simulink model "mdl_VD_st5dofModelFriction_ConstantSpeed"  (R2019b)
settings: Solver=ode4  StartTime=0.0  StopTime=50  FixedStep=deltaT  RelTol=1e-4  EnableMultiTasking=on
values from neighbouring files (symbols this model uses):
  friction_coefficient = [0.9, 0.9]    [script_test_mdl_VD_st5dofModel.m]    (also in script_test_mdl_VD_st5dofModelFriction.m; script_test_mdl_VD_st5dofModelFriction_ConstantSpeed.m)
  Period = 3    [script_test_mdl_VD_BicycleModel.m]    (also in script_test_mdl_VD_st5dofModel.m; script_test_mdl_VD_st5dofModelFriction.m; script_test_mdl_VD_st5dofModelFriction_ConstantSpeed.m)
  steering_amplitude = 2*pi/180    (= 0.0349065850399)    [script_test_mdl_VD_st5dofModel.m]    (also in script_test_mdl_VD_st5dofModelFriction.m; script_test_mdl_VD_st5dofModelFriction_ConstantSpeed.m)
undefined symbols (not defined in the file or in its folder): initial, road_properties, vdParam, vehicle
libraries: simulink x5
settings Model: Creator=cbeal  LastModifiedBy=prasa
settings SolverCC: ZeroCrossAlgorithm=Adaptive
settings DataIOCC: SaveFormat=Array  SaveTime=off  ReturnWorkspaceOutputs=off
settings OptimizationCC: ExpressionDepthLimit=2147483647  LifeSpan=inf
settings DebuggingCC: ReadBeforeWriteMsg=DisableAll  WriteAfterWriteMsg=DisableAll  WriteAfterReadMsg=DisableAll  UnderspecifiedInitializationDetection=Classic  MergeDetectMultiDrivingBlocksExec=none  SolverPrmCheckMsg=warning  MultiTaskDSMMsg=none  FcnCallInpInsideContextMsg=warning  StateNameClashWarn=warning  SFUnexpectedBacktrackingDiag=warning  SFNoUnconditionalDefaultTransitionDiag=warning  SFExecutionAtInitializationDiag=none  ArithmeticOperatorsInVariantConditions=warning
settings HardwareCC: ProdBitPerPointer=32  ProdBitPerSizeT=32  ProdBitPerPtrDiffT=32  ProdLargestAtomicFloat=None  ProdIntDivRoundTo=Undefined  ProdEndianess=Unspecified  ProdWordSize=32  ProdHWDeviceType=32-bit Generic
settings ModelReferenceCC: UpdateModelReferenceTargets=IfOutOfDate  PropagateSignalLabelsOutOfModel=off
settings SFSimCC: SFSimEcho=off  SimUseLocalCustomCode=off  CustomCodeUndefinedFunction=UseInterfaceOnly
settings RTWCC: RTWUseLocalCustomCode=off
settings CodeAppCC: StateflowObjectComments=on
settings GRTTargetCC: TargetLangStandard=C89/C90 (ANSI)
settings ConfigComp: CovMetricSettings=dw  CovHtmlReporting=on  CovSaveCumulativeToWorkspaceVar=on  CovSaveSingleToWorkspaceVar=on  CovExternalEMLEnable=off

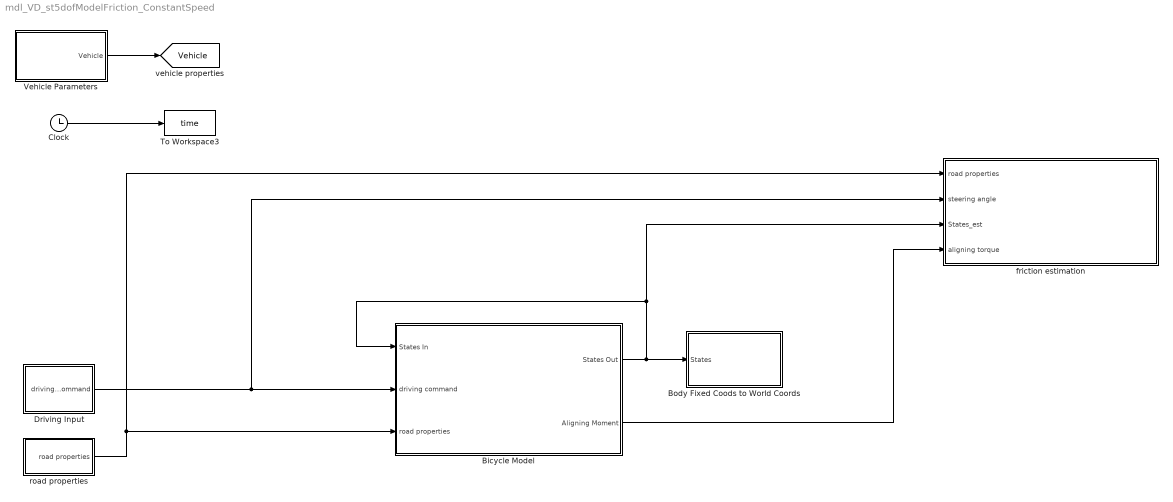
== system mdl_VD_st5dofModelFriction_ConstantSpeed ==
  Bicycle Model : Subsystem
  Body Fixed Coods to World Coords : Subsystem
      mask Display: image('$imagefile'); % Use "Edit Image" on toolstrip to change.
  Clock : Clock
  Driving Input : Subsystem
  To Workspace3 : ToWorkspace  VariableName=time  SampleTime=-1
  Vehicle Parameters : Subsystem  mask{vehicleName='C5 Vette', m=1600, Izz=2500, Iw=1.2, Re=0.32, a=1.3, b=1.3, d=1.5, h_cg=0.42, Ca=[95000; 95000; 110000; 110000], Cx=[65000,65000,65000,65000]}
      mask prompts: vehicleName "Name of Vehicle"; m "Mass"; Izz "Yaw Moment of Inertia"; Iw "Wheel Moment of Inertia"; Re "Wheel Effective Radius"; a "CG-Front Axle Distance"; b "CG-Rear Axle Distance"; d "Track Width"; h_cg "CG height"; Ca "Cornering Stiffnesses (x4)"; Cx "Longitudinal Stiffnesses (x4)"
      mask Display: port_label('output',1,vehicleName)
  friction estimation : Subsystem
  road properties : Subsystem
  tag scope: Vehicle=global
  wires:
  Clock/1 -> To Workspace3/1
  Driving Input/1(driving command) -> friction estimation/2(steering angle), Bicycle Model/2(driving command)
  road properties/1(road properties) -> Bicycle Model/3(road properties), friction estimation/1(road properties)
  Vehicle Parameters/1(Vehicle) -> [Vehicle]
  Bicycle Model/1(States Out) -> Bicycle Model/1(States In), friction estimation/3(States_est), Body Fixed Coods to World Coords/1(States)
  Bicycle Model/2(Aligning Moment) -> friction estimation/4(aligning torque)

== system mdl_VD_st5dofModelFriction_ConstantSpeed/Bicycle Model ==
  States In : Inport
  driving command : Inport  Port=2
  road properties : Inport  Port=3
  Brush Model : Subsystem
  Normal Forces : Subsystem
      mask Display: image('$imagefile'); % Use "Edit Image" on toolstrip to change.
  Slips : Subsystem
      mask Display: image('$imagefile'); % Use "Edit Image" on toolstrip to change.
  Vehicle Body Newtonian Dynamics : Subsystem
      mask Display: image('$imagefile'); % Use "Edit Image" on toolstrip to change.
  States Out : Outport
  Aligning Moment : Outport  Port=2
  wires:
  road properties/1 -> Normal Forces/2(road geometry), Brush Model/3(Road Friction), Vehicle Body Newtonian Dynamics/4(Road Geometry)
  Normal Forces/1(Normal Forces) -> Brush Model/2(Normal Forces)  "Normal Forces"
  States In/1 -> Slips/1(Speeds), Normal Forces/1(accelerations), Vehicle Body Newtonian Dynamics/3(States_IN)
  Vehicle Body Newtonian Dynamics/1(States_Out) -> States Out/1
  Brush Model/1(Aligning Moment) -> Aligning Moment/1
  Slips/1(Slips) -> Brush Model/1(Slips)  "Slips"
  Brush Model/2(Tire Forces) -> Vehicle Body Newtonian Dynamics/1(Tire Forces)
  driving command/1 -> Slips/2(steering angle), Vehicle Body Newtonian Dynamics/2(Driving Command)

== system mdl_VD_st5dofModelFriction_ConstantSpeed/Body Fixed Coods to World Coords ==
  States : Inport
  Bus Creator1 : BusCreator  Inputs=3
  Bus Selector4 : BusSelector  OutputSignals=speeds.Vx,speeds.Vy,speeds.r
  Integrator_East : Integrator  InitialCondition=initial.east
  Integrator_North : Integrator  InitialCondition=initial.north
  Integrator_Psi : Integrator  InitialCondition=initial.heading
  Product{4..7} (4 alike) : Product  SaturateOnIntegerOverflow=on  OutDataTypeStr=Inherit: Same as first input
  Sum : Sum  Inputs=+-  SaturateOnIntegerOverflow=on
  Sum1 : Sum  SaturateOnIntegerOverflow=on
  To Workspace6 : ToWorkspace  VariableName=pose  SampleTime=-1
  Trigonometric Function2 : Trigonometry
  Trigonometric Function3 : Trigonometry  Operator=cos
  wires:
  Bus Creator1/1 -> To Workspace6/1
  Product4/1 -> Sum1/1
  Product6/1 -> Sum/2
  Product7/1 -> Sum1/2
  Trigonometric Function2/1 -> Product4/2, Product6/2
  Integrator_Psi/1 -> Bus Creator1/3, Trigonometric Function3/1, Trigonometric Function2/1  "PSI"
  Sum1/1 -> Integrator_North/1
  Sum/1 -> Integrator_East/1
  Trigonometric Function3/1 -> Product5/2, Product7/2
  Integrator_East/1 -> Bus Creator1/1  "East"
  Product5/1 -> Sum/1
  Integrator_North/1 -> Bus Creator1/2  "North"
  Bus Selector4/1 -> Product4/1, Product5/1  "<Vx>"
  Bus Selector4/3 -> Integrator_Psi/1  "<r>"
  Bus Selector4/2 -> Product7/1, Product6/1  "<Vy>"
  States/1 -> Bus Selector4/1

== system mdl_VD_st5dofModelFriction_ConstantSpeed/Driving Input ==
  Bus Creator1 : BusCreator  Inputs=1
  Mux2 : Mux  Inputs=2
  Product : Product  SaturateOnIntegerOverflow=on  OutDataTypeStr=Inherit: Same as first input
  Rear Steering : Constant  Value=0
  Sine Wave : Sin  Amplitude=steering_amplitude  Frequency=2*pi/Period  SampleTime=0
  Step : Step  Time=0  SampleTime=0
  Step1 : Step  Time=Period  SampleTime=0
  Sum : Sum  Inputs=|+-  SaturateOnIntegerOverflow=on
  To Workspace3 : ToWorkspace  VariableName=delta  SampleTime=-1
  driving command : Outport
  wires:
  Mux2/1 -> To Workspace3/1, Bus Creator1/1  "steering angle"
  Bus Creator1/1 -> driving command/1
  Step1/1 -> Sum/2
  Sine Wave/1 -> Product/2
  Sum/1 -> Product/1
  Product/1 -> Mux2/1
  Step/1 -> Sum/1
  Rear Steering/1 -> Mux2/2

== system mdl_VD_st5dofModelFriction_ConstantSpeed/Vehicle Parameters ==
  Bus Creator1 : BusCreator  Inputs=11
  Constant : Constant  Value=vehicle.m
  Constant1 : Constant  Value=vehicle.Izz
  Constant13 : Constant  Value=vehicle.Re
  Constant14 : Constant  Value=vehicle.h_cg
  Constant2 : Constant  Value=vehicle.L
  Constant3 : Constant  Value=vehicle.d
  Constant4 : Constant  Value=vehicle.b
  Constant5 : Constant  Value=vehicle.a
  Constant7 : Constant  Value=vehicle.Ca
  Constant8 : Constant  Value=vehicle.Cx
  Constant9 : Constant  Value=vehicle.Iw
  Vehicle : Outport
  wires:
  Bus Creator1/1 -> Vehicle/1
  Constant/1 -> Bus Creator1/1  "m"
  Constant1/1 -> Bus Creator1/2  "Izz"
  Constant9/1 -> Bus Creator1/3  "Iw"
  Constant13/1 -> Bus Creator1/4  "Re"
  Constant2/1 -> Bus Creator1/6  "L"
  Constant14/1 -> Bus Creator1/9  "h_cg"
  Constant7/1 -> Bus Creator1/10  "Ca"
  Constant8/1 -> Bus Creator1/11  "Cx"
  Constant5/1 -> Bus Creator1/5  "a"
  Constant3/1 -> Bus Creator1/8  "d"
  Constant4/1 -> Bus Creator1/7  "b"

== system mdl_VD_st5dofModelFriction_ConstantSpeed/friction estimation ==
  road properties : Inport
  steering angle : Inport  Port=2
  States_est : Inport  Port=3
  aligning torque : Inport  Port=4
  Bus Selector1 : BusSelector  OutputSignals=road friction,road geometry
  Bus Selector2 : BusSelector  OutputSignals=steering angle
  Friction Coefficients Estimate : Subsystem
  Noise Models : Subsystem
  Normal Forces : Subsystem
      mask Display: image('$imagefile'); % Use "Edit Image" on toolstrip to change.
  Slip Angle : Subsystem
      mask Display: image('$imagefile'); % Use "Edit Image" on toolstrip to change.
  To Workspace1 : ToWorkspace  VariableName=friction_coefficients_estimate  SampleTime=-1
  fric est Calculate Xis : Subsystem
  wires:
  States_est/1 -> Noise Models/1(" States")
  Bus Selector2/1 -> Slip Angle/2(delta)  "<steering angle>"
  aligning torque/1 -> Friction Coefficients Estimate/1(Mz)
  fric est Calculate Xis/1(fric est coefficients) -> Friction Coefficients Estimate/2(fric est coefficients)
  Normal Forces/1(Normal Forces) -> Friction Coefficients Estimate/3(fric est Normal Forces)
  Bus Selector1/2 -> Normal Forces/2(road geometry)  "<road geometry>"
  Friction Coefficients Estimate/1(friction coefficients Estimate) -> To Workspace1/1  "friction_coeffs_estimate"
  Bus Selector1/1 -> fric est Calculate Xis/2(friction coefficients)  "<road friction>"
  road properties/1 -> Bus Selector1/1
  Slip Angle/1(Slip Angles) -> fric est Calculate Xis/1(Slip Angles est)
  Noise Models/1(Speeds) -> Slip Angle/1(Speeds)
  steering angle/1 -> Bus Selector2/1
  Noise Models/2(Accelerations) -> Normal Forces/1(accelerations)

== system mdl_VD_st5dofModelFriction_ConstantSpeed/road properties ==
  Bus Creator1 : BusCreator  Inputs=3
  Bus Creator2 : BusCreator  Inputs=2
  Constant1 : Constant  Value=road_properties.grade
  Constant19 : Constant  Value=road_properties.bank_angle
  Constant3 : Constant  Value=0
  Constant4 : Constant  Value=friction_coefficient
  road properties : Outport
  wires:
  Constant1/1 -> Bus Creator1/2  "grade"
  Constant19/1 -> Bus Creator1/1  "banking angle"
  Constant3/1 -> Bus Creator1/3  "Curvature"
  Constant4/1 -> Bus Creator2/2  "road friction"
  Bus Creator2/1 -> road properties/1  "road properties"
  Bus Creator1/1 -> Bus Creator2/1  "road geometry"

== system mdl_VD_st5dofModelFriction_ConstantSpeed/Bicycle Model/Brush Model ==
  Slips : Inport
  Normal Forces : Inport  Port=2
  Road Friction : Inport  Port=3
  Aligning Moment_Brush Model : Subsystem
      mask Display: image('$imagefile'); % Use "Edit Image" on toolstrip to change.
  Tire Forces_Brush Model : Subsystem
      mask Display: image('$imagefile'); % Use "Edit Image" on toolstrip to change.
  Aligning Moment : Outport
  Tire Forces : Outport  Port=2
  wires:
  Road Friction/1 -> Aligning Moment_Brush Model/3(Friction Coefficients), Tire Forces_Brush Model/3(road friction)
  Tire Forces_Brush Model/1(Tire Forces) -> Tire Forces/1  "Tire Forces"
  Aligning Moment_Brush Model/1(Aligning Moment) -> Aligning Moment/1  "Aligning Moment"
  Normal Forces/1 -> Tire Forces_Brush Model/2(Normal Forces), Aligning Moment_Brush Model/2(Normal Forces)
  Slips/1 -> Tire Forces_Brush Model/1(Slips), Aligning Moment_Brush Model/1(Slip Angles)

== system mdl_VD_st5dofModelFriction_ConstantSpeed/Bicycle Model/Normal Forces ==
  accelerations : Inport
  road geometry : Inport  Port=2
  Front : Sum  Inputs=+-
  Mux : Mux  Inputs=2
  Normal Force Longitudinal Transfer : Subsystem
      mask Display: image('$imagefile'); % Use "Edit Image" on toolstrip to change.
  Normal Force Static : Subsystem
  Rear : Sum
  Normal Forces : Outport
  wires:
  Mux/1 -> Normal Forces/1
  Front/1 -> Mux/1
  Rear/1 -> Mux/2
  Normal Force Static/2(Static Rear) -> Rear/1
  Normal Force Static/1(Static Front) -> Front/1
  road geometry/1 -> Normal Force Static/1(road geometry)
  Normal Force Longitudinal Transfer/1(Long Transfer) -> Front/2, Rear/2
  accelerations/1 -> Normal Force Longitudinal Transfer/1(Accelerations)

== system mdl_VD_st5dofModelFriction_ConstantSpeed/Bicycle Model/Slips ==
  Speeds : Inport
  steering angle : Inport  Port=2
  Bus Creator : BusCreator  Inputs=2
  Bus Selector1 : BusSelector  OutputSignals=speeds
  Bus Selector2 : BusSelector  OutputSignals=steering angle
  Slip Angle : Subsystem
      mask Display: image('$imagefile'); % Use "Edit Image" on toolstrip to change.
  To Workspace : ToWorkspace  VariableName=alpha  SampleTime=-1
  To Workspace4 : ToWorkspace  VariableName=kappa  SampleTime=-1
  Wheel Slip Ratio : Subsystem
      mask Display: image('$imagefile'); % Use "Edit Image" on toolstrip to change.
  Slips : Outport
  wires:
  Slip Angle/1(Slip Angles) -> Bus Creator/1, To Workspace/1  "Slip Angles"
  Bus Selector2/1 -> Wheel Slip Ratio/1(delta), Slip Angle/2(delta)  "<steering angle>"
  Wheel Slip Ratio/1(Wheel Slips) -> To Workspace4/1, Bus Creator/2  "Wheel Slips"
  Bus Selector1/1 -> Slip Angle/1(Speeds), Wheel Slip Ratio/2(Speeds)  "<speeds>"
  Bus Creator/1 -> Slips/1
  Speeds/1 -> Bus Selector1/1
  steering angle/1 -> Bus Selector2/1

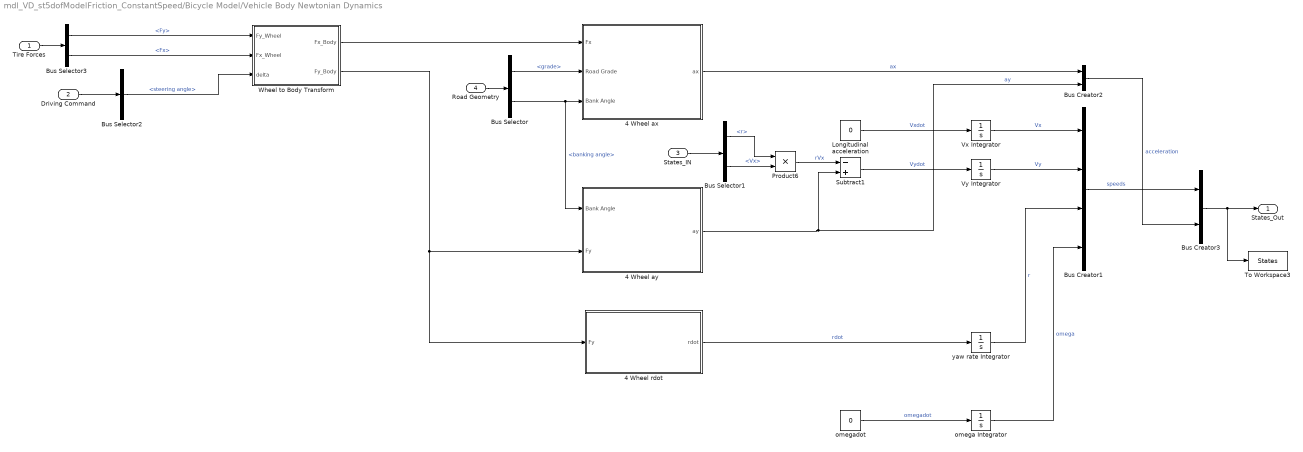
== system mdl_VD_st5dofModelFriction_ConstantSpeed/Bicycle Model/Vehicle Body Newtonian Dynamics ==
  Tire Forces : Inport
  Driving Command : Inport  Port=2
  States_IN : Inport  Port=3
  Road Geometry : Inport  Port=4
  4 Wheel ax : Subsystem
  4 Wheel ay : Subsystem
  4 Wheel rdot : Subsystem
  Bus Creator1 : BusCreator  Inputs=4
  Bus Creator2 : BusCreator  Inputs=2
  Bus Creator3 : BusCreator  Inputs=2
  Bus Selector : BusSelector  OutputSignals=road geometry.grade,road geometry.banking angle
  Bus Selector1 : BusSelector  OutputSignals=speeds.r,speeds.Vx
  Bus Selector2 : BusSelector  OutputSignals=steering angle
  Bus Selector3 : BusSelector  OutputSignals=Fy,Fx
  Longitudinal acceleration : Constant  Value=0
  Product6 : Product  RndMeth=Zero
  Subtract1 : Sum  Inputs=-+
  To Workspace3 : ToWorkspace  VariableName=States  SampleTime=-1
  Vx Integrator : Integrator  InitialCondition=initial.longitudinalSpeed
  Vy Integrator : Integrator
  Wheel to Body Transform : Subsystem
  omega Integrator : Integrator  InitialCondition=initial.wheelSpeeds
  omegadot : Constant  Value=0
  yaw rate Integrator : Integrator
  States_Out : Outport
  wires:
  omegadot/1 -> omega Integrator/1  "omegadot"
  yaw rate Integrator/1 -> Bus Creator1/3  "r"
  Vy Integrator/1 -> Bus Creator1/2  "Vy"
  Vx Integrator/1 -> Bus Creator1/1  "Vx"
  omega Integrator/1 -> Bus Creator1/4  "omega"
  Bus Creator2/1 -> Bus Creator3/2  "acceleration"
  Product6/1 -> Subtract1/1  "rVx"
  Longitudinal acceleration/1 -> Vx Integrator/1  "Vxdot"
  Bus Selector/1 -> 4 Wheel ax/2(Road Grade)  "<grade>"
  Wheel to Body Transform/2(Fy_Body) -> 4 Wheel rdot/1(Fy), 4 Wheel ay/2(Fy)
  Wheel to Body Transform/1(Fx_Body) -> 4 Wheel ax/1("Fx ")
  4 Wheel rdot/1(rdot) -> yaw rate Integrator/1  "rdot"
  4 Wheel ay/1(ay) -> Bus Creator2/2, Subtract1/2  "ay"
  4 Wheel ax/1(ax) -> Bus Creator2/1  "ax"
  Bus Creator1/1 -> Bus Creator3/1  "speeds"
  Bus Selector/2 -> 4 Wheel ay/1(Bank Angle), 4 Wheel ax/3(Bank Angle)  "<banking angle>"
  Road Geometry/1 -> Bus Selector/1
  Bus Selector2/1 -> Wheel to Body Transform/3(delta)  "<steering angle>"
  States_IN/1 -> Bus Selector1/1
  Bus Selector1/2 -> Product6/2  "<Vx>"
  Bus Selector1/1 -> Product6/1  "<r>"
  Tire Forces/1 -> Bus Selector3/1
  Bus Selector3/2 -> Wheel to Body Transform/2(Fx_Wheel)  "<Fx>"
  Bus Selector3/1 -> Wheel to Body Transform/1(Fy_Wheel)  "<Fy>"
  Driving Command/1 -> Bus Selector2/1
  Bus Creator3/1 -> To Workspace3/1, States_Out/1
  Subtract1/1 -> Vy Integrator/1  "Vydot"

== system mdl_VD_st5dofModelFriction_ConstantSpeed/friction estimation/Friction Coefficients Estimate ==
  Mz : Inport
  fric est coefficients : Inport  Port=2
  fric est Normal Forces : Inport  Port=3
  Demux1 : Demux
  Divide : Product  Inputs=*/
  Estimate Friction Force : M-S-Function  FunctionName=sfcn_estimateFrictionForce_Bicycle
  To Workspace5 : ToWorkspace  VariableName=frictionalForce_est  SampleTime=-1
  friction coefficients Estimate : Outport
  wires:
  fric est coefficients/1 -> Demux1/1
  Estimate Friction Force/1 -> Divide/1, To Workspace5/1
  Mz/1 -> Estimate Friction Force/1
  Demux1/1 -> Estimate Friction Force/2  "Xi1"
  Demux1/2 -> Estimate Friction Force/3  "Xi2"
  Demux1/3 -> Estimate Friction Force/4  "Xi3"
  Demux1/4 -> Estimate Friction Force/5  "Xi4"
  fric est Normal Forces/1 -> Divide/2
  Divide/1 -> friction coefficients Estimate/1

== system mdl_VD_st5dofModelFriction_ConstantSpeed/friction estimation/Noise Models ==
  " States" : Inport
  Bus Creator1 : BusCreator  Inputs=3
  Bus Creator2 : BusCreator  Inputs=2
  Bus Creator3 : BusCreator  Inputs=2
  Bus Selector1 : BusSelector  OutputSignals=acceleration,speeds
  Bus Selector2 : BusSelector  OutputSignals=Vx,Vy,r
  Bus Selector3 : BusSelector  OutputSignals=ax,ay
  GPS Noise Function : MATLAB Function  TreatAsAtomicUnit=on
  IMU Noise Function : MATLAB Function  TreatAsAtomicUnit=on
  Sampling Time : Constant  Value=vdParam.sampling_time_gps
  Sampling Time1 : Constant  Value=vdParam.sampling_time_imu
  Speeds : Outport
  Accelerations : Outport  Port=2
  wires:
  Bus Selector2/3 -> GPS Noise Function/3(r)  "<r>"
  Bus Selector1/2 -> Bus Selector2/1  "<speeds>"
  Bus Selector2/2 -> GPS Noise Function/2(v_y)  "<Vy>"
  Bus Selector2/1 -> GPS Noise Function/1(v_x)  "<Vx>"
  Bus Creator1/1 -> Bus Creator3/2, Speeds/1  "speeds"
  Bus Selector3/1 -> IMU Noise Function/1(a_x)  "<ax>"
  Bus Selector3/2 -> IMU Noise Function/2(a_y)  "<ay>"
  Bus Selector1/1 -> Bus Selector3/1  "<acceleration>"
  GPS Noise Function/3(r_out) -> Bus Creator1/3  "r"
  Bus Creator2/1 -> Bus Creator3/1  "acceleration"
  Sampling Time/1 -> GPS Noise Function/4(sampling_time)
  GPS Noise Function/1(v_x_out) -> Bus Creator1/1  "Vx"
  GPS Noise Function/2(v_y_out) -> Bus Creator1/2  "Vy"
  IMU Noise Function/2(a_y_out) -> Bus Creator2/2  "ay"
  IMU Noise Function/1(a_x_out) -> Bus Creator2/1  "ax"
  Sampling Time1/1 -> IMU Noise Function/3(sampling_time)
  " States"/1 -> Bus Selector1/1
  Bus Creator3/1 -> Accelerations/1

== system mdl_VD_st5dofModelFriction_ConstantSpeed/friction estimation/Normal Forces ==
  accelerations : Inport
  road geometry : Inport  Port=2
  Front : Sum  Inputs=+-
  Mux : Mux  Inputs=2
  Normal Force Longitudinal Transfer : Subsystem
      mask Display: image('$imagefile'); % Use "Edit Image" on toolstrip to change.
  Normal Force Static : Subsystem
  Rear : Sum
  Normal Forces : Outport
  wires:
  Mux/1 -> Normal Forces/1
  Front/1 -> Mux/1
  Rear/1 -> Mux/2
  Normal Force Static/2(Static Rear) -> Rear/1
  Normal Force Static/1(Static Front) -> Front/1
  road geometry/1 -> Normal Force Static/1(road geometry)
  Normal Force Longitudinal Transfer/1(Long Transfer) -> Front/2, Rear/2
  accelerations/1 -> Normal Force Longitudinal Transfer/1(Accelerations)

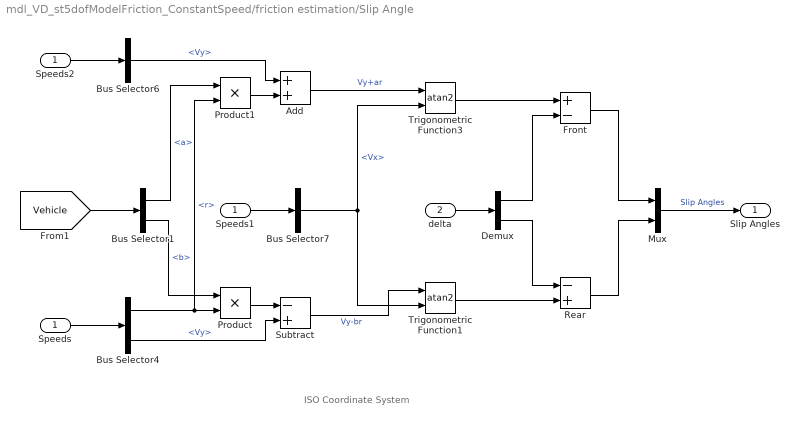
== system mdl_VD_st5dofModelFriction_ConstantSpeed/friction estimation/Slip Angle ==
  note: ISO Coordinate System
  Speeds : Inport
  delta : Inport  Port=2
  Add : Sum
  Bus Selector1 : BusSelector  OutputSignals=a,b
  Bus Selector4 : BusSelector  OutputSignals=r,Vy
  Bus Selector6 : BusSelector  OutputSignals=Vy
  Bus Selector7 : BusSelector  OutputSignals=Vx
  Demux : Demux  Outputs=2
  Front : Sum  Inputs=+-
  Mux : Mux  Inputs=2
  Product : Product  RndMeth=Zero
  Product1 : Product  RndMeth=Zero
  Rear : Sum  Inputs=-+
  Speeds1 : InportShadow
  Speeds2 : InportShadow
  Subtract : Sum  Inputs=-+
  Trigonometric Function1 : Trigonometry  Operator=atan2
  Trigonometric Function3 : Trigonometry  Operator=atan2
  Slip Angles : Outport
  wires:
  Speeds1/1 -> Bus Selector7/1
  Bus Selector4/1 -> Product1/2, Product/2  "<r>"
  Demux/1 -> Front/2
  Subtract/1 -> Trigonometric Function1/1  "Vy-br"
  Trigonometric Function1/1 -> Rear/2
  delta/1 -> Demux/1
  Rear/1 -> Mux/2
  Demux/2 -> Rear/1
  Add/1 -> Trigonometric Function3/1  "Vy+ar"
  [Vehicle] -> Bus Selector1/1
  Product/1 -> Subtract/1
  Mux/1 -> Slip Angles/1  "Slip Angles"
  Bus Selector1/2 -> Product/1  "<b>"
  Front/1 -> Mux/1
  Bus Selector1/1 -> Product1/1  "<a>"
  Trigonometric Function3/1 -> Front/1
  Product1/1 -> Add/2
  Bus Selector7/1 -> Trigonometric Function3/2, Trigonometric Function1/2  "<Vx>"
  Speeds2/1 -> Bus Selector6/1
  Bus Selector4/2 -> Subtract/2  "<Vy>"
  Bus Selector6/1 -> Add/1  "<Vy>"
  Speeds/1 -> Bus Selector4/1

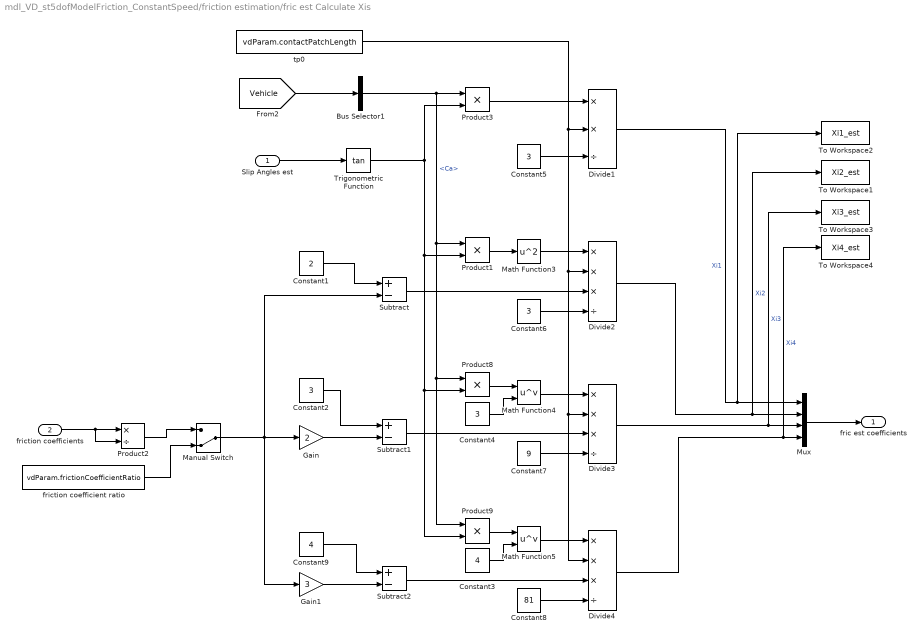
== system mdl_VD_st5dofModelFriction_ConstantSpeed/friction estimation/fric est Calculate Xis ==
  Slip Angles est : Inport
  friction coefficients : Inport  Port=2
  Bus Selector1 : BusSelector  OutputSignals=Ca
  Constant1 : Constant  Value=2
  Constant{2,4..6} (4 alike) : Constant  Value=3
  Constant3 : Constant  Value=4
  Constant7 : Constant  Value=9
  Constant8 : Constant  Value=81
  Constant9 : Constant  Value=4
  Divide1 : Product  Inputs=**/
  Divide2 : Product  Inputs=***/
  Divide3 : Product  Inputs=***/
  Divide4 : Product  Inputs=***/
  Gain : Gain  Gain=2
  Gain1 : Gain  Gain=3
  Manual Switch : ManualSwitch  CurrentSetting=0
  Math Function3 : Math  Operator=square  SaturateOnIntegerOverflow=on
  Math Function4 : Math  Operator=pow  SignedPower=off  SaturateOnIntegerOverflow=on
  Math Function5 : Math  Operator=pow  SignedPower=off  SaturateOnIntegerOverflow=on
  Mux : Mux
  Product{1,3,8..9} (4 alike) : Product  RndMeth=Zero
  Product2 : Product  Inputs=*/  RndMeth=Zero
  Subtract : Sum  Inputs=+-
  Subtract1 : Sum  Inputs=+-
  Subtract2 : Sum  Inputs=+-
  To Workspace1 : ToWorkspace  VariableName=Xi2_est  SampleTime=-1
  To Workspace2 : ToWorkspace  VariableName=Xi1_est  SampleTime=-1
  To Workspace3 : ToWorkspace  VariableName=Xi3_est  SampleTime=-1
  To Workspace4 : ToWorkspace  VariableName=Xi4_est  SampleTime=-1
  Trigonometric Function : Trigonometry  Operator=tan
  friction coefficient ratio : Constant  Value=vdParam.frictionCoefficientRatio
  tp0 : Constant  Value=vdParam.contactPatchLength
  fric est coefficients : Outport
  wires:
  Mux/1 -> fric est coefficients/1
  Trigonometric Function/1 -> Product1/2, Product8/2, Product9/2, Product3/2
  tp0/1 -> Divide4/2, Divide3/2, Divide2/2, Divide1/2
  Bus Selector1/1 -> Product9/1, Product8/1, Product1/1, Product3/1  "<Ca>"
  Constant3/1 -> Math Function5/2
  Constant4/1 -> Math Function4/2
  Math Function3/1 -> Divide2/1
  Product1/1 -> Math Function3/1
  [Vehicle] -> Bus Selector1/1
  Math Function4/1 -> Divide3/1
  Constant5/1 -> Divide1/3
  Slip Angles est/1 -> Trigonometric Function/1
  Math Function5/1 -> Divide4/1
  Product8/1 -> Math Function4/1
  Product9/1 -> Math Function5/1
  Constant7/1 -> Divide3/4
  Product3/1 -> Divide1/1
  Subtract1/1 -> Divide3/3
  Constant1/1 -> Subtract/1
  Constant2/1 -> Subtract1/1
  Manual Switch/1 -> Gain1/1, Subtract/2, Gain/1
  Gain/1 -> Subtract1/2
  Constant9/1 -> Subtract2/1
  Gain1/1 -> Subtract2/2
  Constant6/1 -> Divide2/4
  Subtract/1 -> Divide2/3
  Constant8/1 -> Divide4/4
  Subtract2/1 -> Divide4/3
  Divide1/1 -> To Workspace2/1, Mux/1  "Xi1"
  Divide4/1 -> To Workspace4/1, Mux/4  "Xi4"
  Divide2/1 -> To Workspace1/1, Mux/2  "Xi2"
  Divide3/1 -> To Workspace3/1, Mux/3  "Xi3"
  friction coefficients/1 -> Product2/2, Product2/1
  Product2/1 -> Manual Switch/1
  friction coefficient ratio/1 -> Manual Switch/2

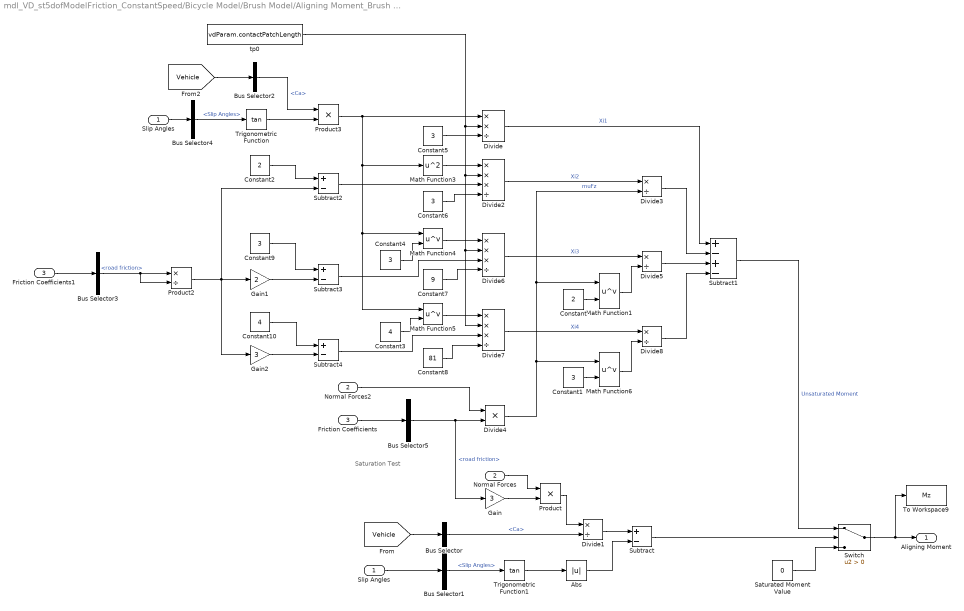
== system mdl_VD_st5dofModelFriction_ConstantSpeed/Bicycle Model/Brush Model/Aligning Moment_Brush Model ==
  note: Saturation Test
  Slip Angles : Inport
  Normal Forces : Inport  Port=2
  Friction Coefficients : Inport  Port=3
  Abs : Abs  ZeroCross=off
  Bus Selector : BusSelector  OutputSignals=Ca
  Bus Selector1 : BusSelector  OutputSignals=Slip Angles
  Bus Selector2 : BusSelector  OutputSignals=Ca
  Bus Selector3 : BusSelector  OutputSignals=road friction
  Bus Selector4 : BusSelector  OutputSignals=Slip Angles
  Bus Selector5 : BusSelector  OutputSignals=road friction
  Constant : Constant  Value=2
  Constant{1,4..6,9} (5 alike) : Constant  Value=3
  Constant10 : Constant  Value=4
  Constant2 : Constant  Value=2
  Constant3 : Constant  Value=4
  Constant7 : Constant  Value=9
  Constant8 : Constant  Value=81
  Divide : Product  Inputs=**/
  Divide{1,3,5,8} (4 alike) : Product  Inputs=*/
  Divide2 : Product  Inputs=***/
  Divide4 : Product
  Divide6 : Product  Inputs=***/
  Divide7 : Product  Inputs=***/
  Friction Coefficients1 : InportShadow  Port=3
  Gain : Gain  Gain=3
  Gain1 : Gain  Gain=2
  Gain2 : Gain  Gain=3
  Math Function{1,4..6} (4 alike) : Math  Operator=pow  SignedPower=off  SaturateOnIntegerOverflow=on
  Math Function3 : Math  Operator=square  SaturateOnIntegerOverflow=on
  Normal Forces2 : InportShadow  Port=2
  Product : Product  RndMeth=Zero
  Product2 : Product  Inputs=*/  RndMeth=Zero
  Product3 : Product  RndMeth=Zero
  Saturated Moment Value : Constant  Value=0
  "Slip Angles " : InportShadow
  Subtract{,2..4} (4 alike) : Sum  Inputs=+-
  Subtract1 : Sum  Inputs=+-+-
  Switch : Switch  Criteria=u2 > Threshold
  To Workspace9 : ToWorkspace  VariableName=Mz  SampleTime=-1
  Trigonometric Function : Trigonometry  Operator=tan
  Trigonometric Function1 : Trigonometry  Operator=tan
  tp0 : Constant  Value=vdParam.contactPatchLength
  Aligning Moment : Outport  VectorParamsAs1DForOutWhenUnconnected=off
  wires:
  Product/1 -> Divide1/1
  Switch/1 -> To Workspace9/1, Aligning Moment/1
  Normal Forces2/1 -> Divide4/1
  Abs/1 -> Subtract/2
  Subtract/1 -> Switch/2
  Saturated Moment Value/1 -> Switch/3
  Bus Selector/1 -> Divide1/2  "<Ca>"
  [Vehicle] -> Bus Selector/1
  Divide1/1 -> Subtract/1
  Normal Forces/1 -> Product/1
  Gain/1 -> Product/2
  Trigonometric Function1/1 -> Abs/1
  Slip Angles/1 -> Bus Selector4/1
  Subtract1/1 -> Switch/1  "Unsaturated Moment"
  "Slip Angles "/1 -> Bus Selector1/1
  Divide4/1 -> Divide3/2, Math Function1/1, Math Function6/1  "muFz"
  Constant/1 -> Math Function1/2
  [Vehicle] -> Bus Selector2/1
  Bus Selector2/1 -> Product3/1  "<Ca>"
  Constant3/1 -> Math Function5/2
  Constant4/1 -> Math Function4/2
  Trigonometric Function/1 -> Product3/2
  Product3/1 -> Math Function3/1, Math Function4/1, Math Function5/1, Divide/1
  tp0/1 -> Divide/2, Divide2/2, Divide7/2, Divide6/2
  Constant5/1 -> Divide/3
  Math Function3/1 -> Divide2/1
  Constant7/1 -> Divide6/4
  Math Function4/1 -> Divide6/1
  Math Function5/1 -> Divide7/1
  Constant6/1 -> Divide2/4
  Constant8/1 -> Divide7/4
  Divide3/1 -> Subtract1/2
  Constant1/1 -> Math Function6/2
  Divide8/1 -> Subtract1/4
  Divide5/1 -> Subtract1/3
  Math Function6/1 -> Divide8/2
  Math Function1/1 -> Divide5/2
  Bus Selector5/1 -> Gain/1, Divide4/2  "<road friction>"
  Divide/1 -> Subtract1/1  "Xi1"
  Divide7/1 -> Divide8/1  "Xi4"
  Divide2/1 -> Divide3/1  "Xi2"
  Divide6/1 -> Divide5/1  "Xi3"
  Gain2/1 -> Subtract4/2
  Product2/1 -> Gain2/1, Subtract2/2, Gain1/1
  Constant9/1 -> Subtract3/1
  Subtract3/1 -> Divide6/3
  Constant10/1 -> Subtract4/1
  Constant2/1 -> Subtract2/1
  Subtract2/1 -> Divide2/3
  Subtract4/1 -> Divide7/3
  Gain1/1 -> Subtract3/2
  Bus Selector4/1 -> Trigonometric Function/1  "<Slip Angles>"
  Bus Selector1/1 -> Trigonometric Function1/1  "<Slip Angles>"
  Bus Selector3/1 -> Product2/2, Product2/1  "<road friction>"
  Friction Coefficients1/1 -> Bus Selector3/1
  Friction Coefficients/1 -> Bus Selector5/1

== system mdl_VD_st5dofModelFriction_ConstantSpeed/Bicycle Model/Brush Model/Tire Forces_Brush Model ==
  note: ISO Coordinate System
  note: [1] J. Svendenius, “Tire Modeling and Friction Estimation,” Control , p. 194, 2007. chapter2.4 and chapter4
      | [2] M. Kissai et al. , “A new linear tire model with varying parameters To cite this version : HAL Id : hal-01690792 A New Linear Tire Model With Varying Parameters,” 2018.
  Slips : Inport
  Normal Forces : Inport  Port=2
  road friction : Inport  Port=3
  Bus Selector2 : BusSelector  OutputSignals=road friction
  Constant3 : Constant
  Switch1 : Switch  Threshold=1  ZeroCross=off
  Wheel Forces : Subsystem
  tire slip : Subsystem
  Tire Forces : Outport
  wires:
  tire slip/1(sigma_x) -> Wheel Forces/3(sigma_x)
  Normal Forces/1 -> tire slip/2(normal force), Wheel Forces/2(normal force)
  tire slip/4(Psi_Tire) -> Switch1/3, Switch1/2
  tire slip/2(sigma_y) -> Wheel Forces/4(sigma_y)
  tire slip/3(sigma) -> Wheel Forces/5(sigma)
  Bus Selector2/1 -> Wheel Forces/1(sliding friction), tire slip/1(peak friction)  "<road friction>"
  Wheel Forces/1(Tire Forces) -> Tire Forces/1
  Constant3/1 -> Switch1/1  "Pure Sliding"
  Switch1/1 -> Wheel Forces/6(Psi_Tire)
  Slips/1 -> tire slip/3(Slips)
  road friction/1 -> Bus Selector2/1

== system mdl_VD_st5dofModelFriction_ConstantSpeed/Bicycle Model/Normal Forces/Normal Force Longitudinal Transfer ==
  Accelerations : Inport
  Bus Selector2 : BusSelector  OutputSignals=m,L,h_cg
  Bus Selector3 : BusSelector  OutputSignals=acceleration.ax
  Compare To Constant : simulink/Logic and Bit Operations/Compare To Constant  relop===  const=1  OutDataTypeStr=boolean
  Constant : Constant  Value=vdParam.longitudinalTransfer
  Delay : Delay  DelayLength=1  InitialCondition=0
  Divide1 : Product  Inputs=/*
  Product1 : Product  RndMeth=Zero
  Product2 : Product  RndMeth=Zero
  Product3 : Product  RndMeth=Zero
  Long Transfer : Outport
  wires:
  Bus Selector2/2 -> Divide1/1  "<L>"
  Product3/1 -> Product1/1
  Bus Selector2/3 -> Divide1/2  "<h_cg>"
  Divide1/1 -> Product1/2
  [Vehicle] -> Bus Selector2/1
  Bus Selector2/1 -> Product2/2  "<m>"
  Delay/1 -> Product2/1
  Product2/1 -> Product3/2
  Product1/1 -> Long Transfer/1
  Accelerations/1 -> Bus Selector3/1
  Compare To Constant/1 -> Product3/1
  Constant/1 -> Compare To Constant/1
  Bus Selector3/1 -> Delay/1  "<ax>"

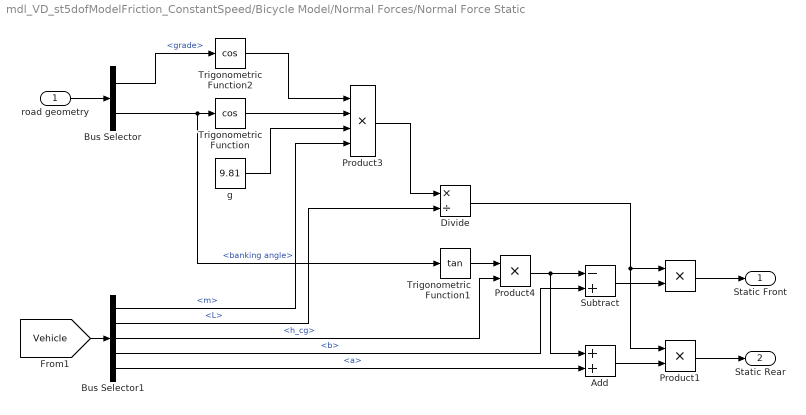
== system mdl_VD_st5dofModelFriction_ConstantSpeed/Bicycle Model/Normal Forces/Normal Force Static ==
  road geometry : Inport
  " " : Product  RndMeth=Zero
  Add : Sum
  Bus Selector : BusSelector  OutputSignals=road geometry.grade,road geometry.banking angle
  Bus Selector1 : BusSelector  OutputSignals=m,L,h_cg,b,a
  Divide : Product  Inputs=*/
  Product1 : Product  RndMeth=Zero
  Product3 : Product  Inputs=4  RndMeth=Zero
  Product4 : Product  RndMeth=Zero
  Subtract : Sum  Inputs=-+
  Trigonometric Function : Trigonometry  Operator=cos
  Trigonometric Function1 : Trigonometry  Operator=tan
  Trigonometric Function2 : Trigonometry  Operator=cos
  g : Constant  Value=9.81
  Static Front : Outport
  Static Rear : Outport  Port=2
  wires:
  Product4/1 -> Add/1, Subtract/1
  Add/1 -> Product1/2
  g/1 -> Product3/3
  [Vehicle] -> Bus Selector1/1
  Bus Selector1/4 -> Subtract/2  "<b>"
  Product3/1 -> Divide/1
  Bus Selector1/1 -> Product3/4  "<m>"
  Trigonometric Function/1 -> Product3/2
  Bus Selector1/5 -> Add/2  "<a>"
  Bus Selector1/3 -> Product4/2  "<h_cg>"
  Trigonometric Function1/1 -> Product4/1
  Divide/1 -> Product1/1, " "/1
  Bus Selector/2 -> Trigonometric Function1/1, Trigonometric Function/1  "<banking angle>"
  Bus Selector1/2 -> Divide/2  "<L>"
  Subtract/1 -> " "/2
  road geometry/1 -> Bus Selector/1
  Product1/1 -> Static Rear/1
  " "/1 -> Static Front/1
  Trigonometric Function2/1 -> Product3/1
  Bus Selector/1 -> Trigonometric Function2/1  "<grade>"

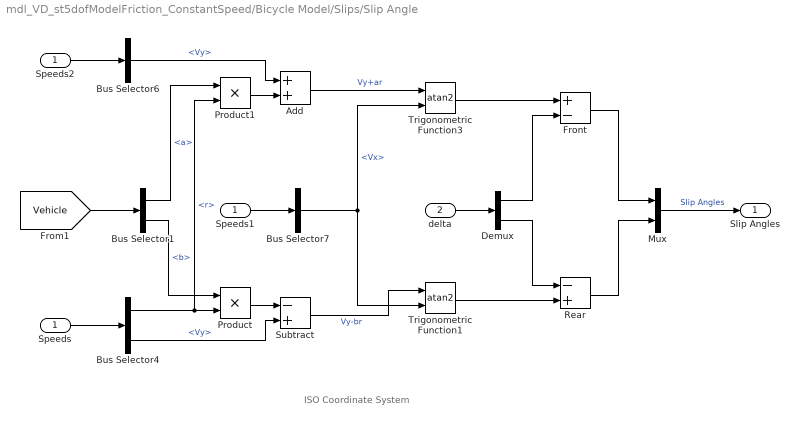
== system mdl_VD_st5dofModelFriction_ConstantSpeed/Bicycle Model/Slips/Slip Angle ==
  note: ISO Coordinate System
  Speeds : Inport
  delta : Inport  Port=2
  Add : Sum
  Bus Selector1 : BusSelector  OutputSignals=a,b
  Bus Selector4 : BusSelector  OutputSignals=r,Vy
  Bus Selector6 : BusSelector  OutputSignals=Vy
  Bus Selector7 : BusSelector  OutputSignals=Vx
  Demux : Demux  Outputs=2
  Front : Sum  Inputs=+-
  Mux : Mux  Inputs=2
  Product : Product  RndMeth=Zero
  Product1 : Product  RndMeth=Zero
  Rear : Sum  Inputs=-+
  Speeds1 : InportShadow
  Speeds2 : InportShadow
  Subtract : Sum  Inputs=-+
  Trigonometric Function1 : Trigonometry  Operator=atan2
  Trigonometric Function3 : Trigonometry  Operator=atan2
  Slip Angles : Outport
  wires:
  Speeds1/1 -> Bus Selector7/1
  Bus Selector4/1 -> Product1/2, Product/2  "<r>"
  Demux/1 -> Front/2
  Subtract/1 -> Trigonometric Function1/1  "Vy-br"
  Trigonometric Function1/1 -> Rear/2
  delta/1 -> Demux/1
  Rear/1 -> Mux/2
  Demux/2 -> Rear/1
  Add/1 -> Trigonometric Function3/1  "Vy+ar"
  [Vehicle] -> Bus Selector1/1
  Product/1 -> Subtract/1
  Mux/1 -> Slip Angles/1  "Slip Angles"
  Bus Selector1/2 -> Product/1  "<b>"
  Front/1 -> Mux/1
  Bus Selector1/1 -> Product1/1  "<a>"
  Trigonometric Function3/1 -> Front/1
  Product1/1 -> Add/2
  Bus Selector7/1 -> Trigonometric Function3/2, Trigonometric Function1/2  "<Vx>"
  Speeds2/1 -> Bus Selector6/1
  Bus Selector4/2 -> Subtract/2  "<Vy>"
  Bus Selector6/1 -> Add/1  "<Vy>"
  Speeds/1 -> Bus Selector4/1

== system mdl_VD_st5dofModelFriction_ConstantSpeed/Bicycle Model/Slips/Wheel Slip Ratio ==
  delta : Inport
  Speeds : Inport  Port=2
  Wheel Slip : Subsystem
  vehicle2tire : Subsystem
  Wheel Slips : Outport
  wires:
  Speeds/1 -> vehicle2tire/2(Speeds), Wheel Slip/2(Speeds)  "Vx,Vy,r,omega"
  delta/1 -> vehicle2tire/1(delta)
  vehicle2tire/1(Vx_tire) -> Wheel Slip/1(Vx_tire)
  Wheel Slip/1(Wheel Slips) -> Wheel Slips/1

== system mdl_VD_st5dofModelFriction_ConstantSpeed/Bicycle Model/Vehicle Body Newtonian Dynamics/4 Wheel ax ==
  "Fx " : Inport
  Road Grade : Inport  Port=2
  Bank Angle : Inport  Port=3
  Add2 : Sum  Inputs=-+
  Bus Selector6 : BusSelector  OutputSignals=m
  Bus Selector7 : BusSelector  OutputSignals=m
  Divide2 : Product  Inputs=/*
  Product10 : Product  Inputs=4  RndMeth=Zero
  Sum of Elements3 : Sum  Inputs=+
  cos : Trigonometry  Operator=cos
  g : Constant  Value=9.81
  sin : Trigonometry
  ax : Outport
  wires:
  [Vehicle] -> Bus Selector6/1
  [Vehicle] -> Bus Selector7/1
  Add2/1 -> Divide2/2
  Bus Selector7/1 -> Divide2/1  "<m>"
  Divide2/1 -> ax/1
  Product10/1 -> Add2/1
  Sum of Elements3/1 -> Add2/2
  Bus Selector6/1 -> Product10/4  "<m>"
  g/1 -> Product10/3
  sin/1 -> Product10/1
  cos/1 -> Product10/2
  Bank Angle/1 -> cos/1
  Road Grade/1 -> sin/1
  "Fx "/1 -> Sum of Elements3/1

== system mdl_VD_st5dofModelFriction_ConstantSpeed/Bicycle Model/Vehicle Body Newtonian Dynamics/4 Wheel ay ==
  Bank Angle : Inport
  Fy : Inport  Port=2
  Add : Sum
  Bus Selector2 : BusSelector  OutputSignals=m
  Bus Selector5 : BusSelector  OutputSignals=m
  Divide1 : Product  Inputs=*/
  Product4 : Product  Inputs=3  RndMeth=Zero
  Sum of Elements : Sum  Inputs=+
  g : Constant  Value=9.81
  sin : Trigonometry
  ay : Outport
  wires:
  [Vehicle] -> Bus Selector2/1
  Fy/1 -> Sum of Elements/1
  Product4/1 -> Add/2
  Add/1 -> Divide1/1
  Bus Selector2/1 -> Divide1/2  "<m>"
  Divide1/1 -> ay/1
  [Vehicle] -> Bus Selector5/1
  g/1 -> Product4/2
  Bus Selector5/1 -> Product4/1  "<m>"
  sin/1 -> Product4/3
  Bank Angle/1 -> sin/1
  Sum of Elements/1 -> Add/1

== system mdl_VD_st5dofModelFriction_ConstantSpeed/Bicycle Model/Vehicle Body Newtonian Dynamics/4 Wheel rdot ==
  Fy : Inport
  Add2 : Sum  Inputs=-+
  Bus Selector1 : BusSelector  OutputSignals=b
  Bus Selector2 : BusSelector  OutputSignals=a
  Bus Selector7 : BusSelector  OutputSignals=Izz
  Divide2 : Product  Inputs=/*
  Product1 : Product  RndMeth=Zero
  Product2 : Product  RndMeth=Zero
  Selector : Selector  InputPortWidth=2  IndexOptions=Index vector (dialog)  Indices=[2]  OutputSizes=1
  Selector1 : Selector  InputPortWidth=2  IndexOptions=Index vector (dialog)  Indices=[1]  OutputSizes=1
  Sum of Elements : Sum  Inputs=+
  Sum of Elements1 : Sum  Inputs=+
  rdot : Outport
  wires:
  Fy/1 -> Selector/1, Selector1/1
  Divide2/1 -> rdot/1
  Bus Selector7/1 -> Divide2/1  "<Izz>"
  Add2/1 -> Divide2/2
  [Vehicle] -> Bus Selector7/1
  [Vehicle] -> Bus Selector1/1
  Selector/1 -> Sum of Elements/1
  Selector1/1 -> Sum of Elements1/1
  Sum of Elements/1 -> Product1/1
  Bus Selector1/1 -> Product1/2  "<b>"
  Product1/1 -> Add2/1
  [Vehicle] -> Bus Selector2/1
  Product2/1 -> Add2/2
  Bus Selector2/1 -> Product2/1  "<a>"
  Sum of Elements1/1 -> Product2/2

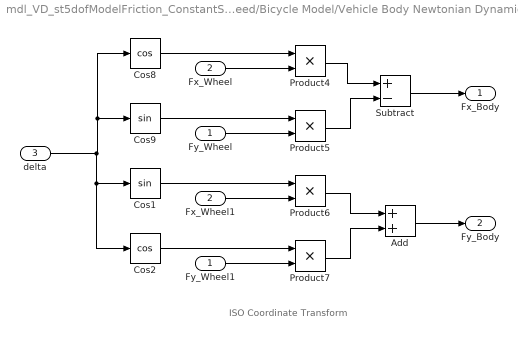
== system mdl_VD_st5dofModelFriction_ConstantSpeed/Bicycle Model/Vehicle Body Newtonian Dynamics/Wheel to Body Transform ==
  note: ISO Coordinate Transform
  Fy_Wheel : Inport
  Fx_Wheel : Inport  Port=2
  delta : Inport  Port=3
  Add : Sum
  Cos1 : Trigonometry
  Cos2 : Trigonometry  Operator=cos
  Cos8 : Trigonometry  Operator=cos
  Cos9 : Trigonometry
  Fx_Wheel1 : InportShadow  Port=2
  Fy_Wheel1 : InportShadow
  Product{4..7} (4 alike) : Product
  Subtract : Sum  Inputs=+-
  Fx_Body : Outport
  Fy_Body : Outport  Port=2
  wires:
  Subtract/1 -> Fx_Body/1
  delta/1 -> Cos8/1, Cos9/1, Cos2/1, Cos1/1
  Cos8/1 -> Product4/1
  Cos9/1 -> Product5/1
  Cos1/1 -> Product6/1
  Cos2/1 -> Product7/1
  Fx_Wheel1/1 -> Product6/2
  Fy_Wheel1/1 -> Product7/2
  Fy_Wheel/1 -> Product5/2
  Fx_Wheel/1 -> Product4/2
  Product4/1 -> Subtract/1
  Product5/1 -> Subtract/2
  Product6/1 -> Add/1
  Product7/1 -> Add/2
  Add/1 -> Fy_Body/1

== system mdl_VD_st5dofModelFriction_ConstantSpeed/friction estimation/Normal Forces/Normal Force Longitudinal Transfer ==
  Accelerations : Inport
  Bus Selector2 : BusSelector  OutputSignals=m,L,h_cg
  Bus Selector3 : BusSelector  OutputSignals=acceleration.ax
  Compare To Constant : simulink/Logic and Bit Operations/Compare To Constant  relop===  const=1  OutDataTypeStr=boolean
  Constant : Constant  Value=vdParam.longitudinalTransfer
  Delay : Delay  DelayLength=1  InitialCondition=0
  Divide1 : Product  Inputs=/*
  Product1 : Product  RndMeth=Zero
  Product2 : Product  RndMeth=Zero
  Product3 : Product  RndMeth=Zero
  Long Transfer : Outport
  wires:
  Bus Selector2/2 -> Divide1/1  "<L>"
  Product3/1 -> Product1/1
  Bus Selector2/3 -> Divide1/2  "<h_cg>"
  Divide1/1 -> Product1/2
  [Vehicle] -> Bus Selector2/1
  Bus Selector2/1 -> Product2/2  "<m>"
  Delay/1 -> Product2/1
  Product2/1 -> Product3/2
  Product1/1 -> Long Transfer/1
  Accelerations/1 -> Bus Selector3/1
  Compare To Constant/1 -> Product3/1
  Constant/1 -> Compare To Constant/1
  Bus Selector3/1 -> Delay/1  "<ax>"

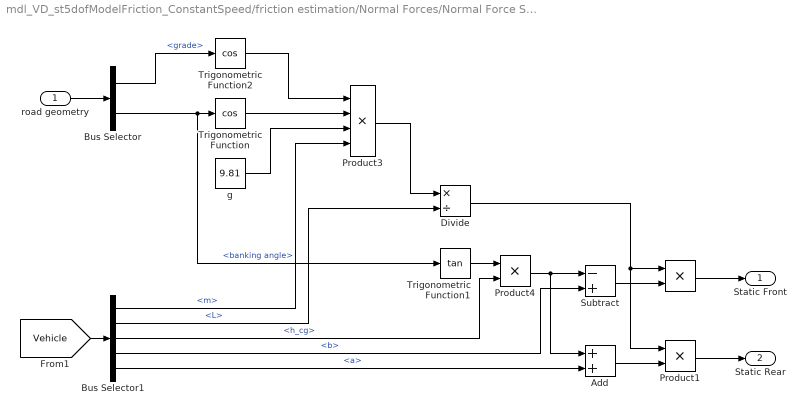
== system mdl_VD_st5dofModelFriction_ConstantSpeed/friction estimation/Normal Forces/Normal Force Static ==
  road geometry : Inport
  " " : Product  RndMeth=Zero
  Add : Sum
  Bus Selector : BusSelector  OutputSignals=grade,banking angle
  Bus Selector1 : BusSelector  OutputSignals=m,L,h_cg,b,a
  Divide : Product  Inputs=*/
  Product1 : Product  RndMeth=Zero
  Product3 : Product  Inputs=4  RndMeth=Zero
  Product4 : Product  RndMeth=Zero
  Subtract : Sum  Inputs=-+
  Trigonometric Function : Trigonometry  Operator=cos
  Trigonometric Function1 : Trigonometry  Operator=tan
  Trigonometric Function2 : Trigonometry  Operator=cos
  g : Constant  Value=9.81
  Static Front : Outport
  Static Rear : Outport  Port=2
  wires:
  Product4/1 -> Add/1, Subtract/1
  Add/1 -> Product1/2
  g/1 -> Product3/3
  [Vehicle] -> Bus Selector1/1
  Bus Selector1/4 -> Subtract/2  "<b>"
  Product3/1 -> Divide/1
  Bus Selector1/1 -> Product3/4  "<m>"
  Trigonometric Function/1 -> Product3/2
  Bus Selector1/5 -> Add/2  "<a>"
  Bus Selector1/3 -> Product4/2  "<h_cg>"
  Trigonometric Function1/1 -> Product4/1
  Divide/1 -> Product1/1, " "/1
  Bus Selector/2 -> Trigonometric Function1/1, Trigonometric Function/1  "<banking angle>"
  Bus Selector1/2 -> Divide/2  "<L>"
  Subtract/1 -> " "/2
  road geometry/1 -> Bus Selector/1
  Product1/1 -> Static Rear/1
  " "/1 -> Static Front/1
  Trigonometric Function2/1 -> Product3/1
  Bus Selector/1 -> Trigonometric Function2/1  "<grade>"

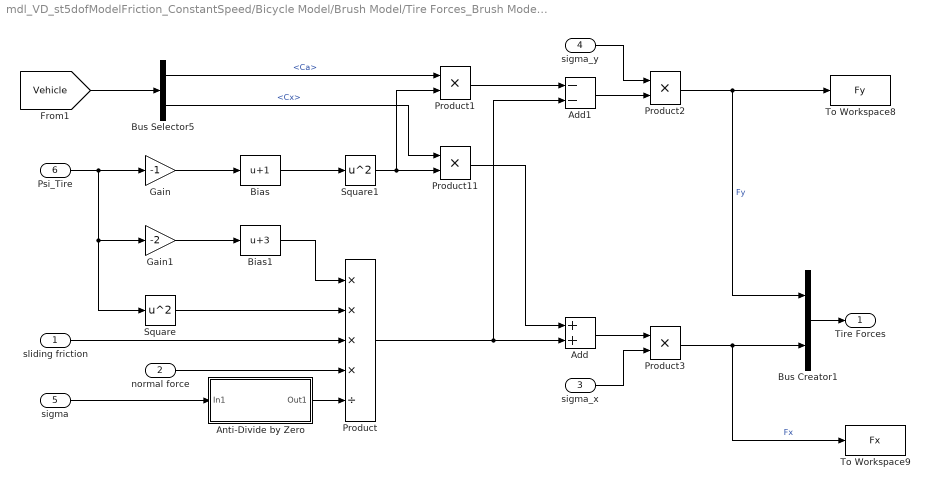
== system mdl_VD_st5dofModelFriction_ConstantSpeed/Bicycle Model/Brush Model/Tire Forces_Brush Model/Wheel Forces ==
  sliding friction : Inport
  normal force : Inport  Port=2
  sigma_x : Inport  Port=3
  sigma_y : Inport  Port=4
  sigma : Inport  Port=5
  Psi_Tire : Inport  Port=6
  Add : Sum
  Add1 : Sum  Inputs=--
  Anti-Divide by Zero : Subsystem
  Bias : Bias  Bias=1
  Bias1 : Bias  Bias=3
  Bus Creator1 : BusCreator  Inputs=2
  Bus Selector5 : BusSelector  OutputSignals=Ca,Cx
  Gain : Gain  Gain=-1
  Gain1 : Gain  Gain=-2
  Product : Product  Inputs=****/
  Product{1..3,11} (4 alike) : Product  RndMeth=Zero
  Square : Math  Operator=square  SignedPower=off  SaturateOnIntegerOverflow=on
  Square1 : Math  Operator=square  SignedPower=off  SaturateOnIntegerOverflow=on
  To Workspace8 : ToWorkspace  VariableName=Fy  SampleTime=-1
  To Workspace9 : ToWorkspace  VariableName=Fx  SampleTime=-1
  Tire Forces : Outport
  wires:
  Product/1 -> Add1/2, Add/2
  Bus Selector5/2 -> Product11/1  "<Cx>"
  [Vehicle] -> Bus Selector5/1
  Gain/1 -> Bias/1
  Gain1/1 -> Bias1/1
  Bias/1 -> Square1/1
  Psi_Tire/1 -> Square/1, Gain1/1, Gain/1
  Square/1 -> Product/2
  Bias1/1 -> Product/1
  sliding friction/1 -> Product/3
  normal force/1 -> Product/4
  sigma/1 -> Anti-Divide by Zero/1(In1)
  Square1/1 -> Product1/2, Product11/2
  Product11/1 -> Add/1
  Bus Selector5/1 -> Product1/1  "<Ca>"
  Product1/1 -> Add1/1
  Add1/1 -> Product2/2
  sigma_y/1 -> Product2/1
  sigma_x/1 -> Product3/2
  Add/1 -> Product3/1
  Bus Creator1/1 -> Tire Forces/1
  Product2/1 -> Bus Creator1/1, To Workspace8/1  "Fy"
  Product3/1 -> To Workspace9/1, Bus Creator1/2  "Fx"
  Anti-Divide by Zero/1(Out1) -> Product/5

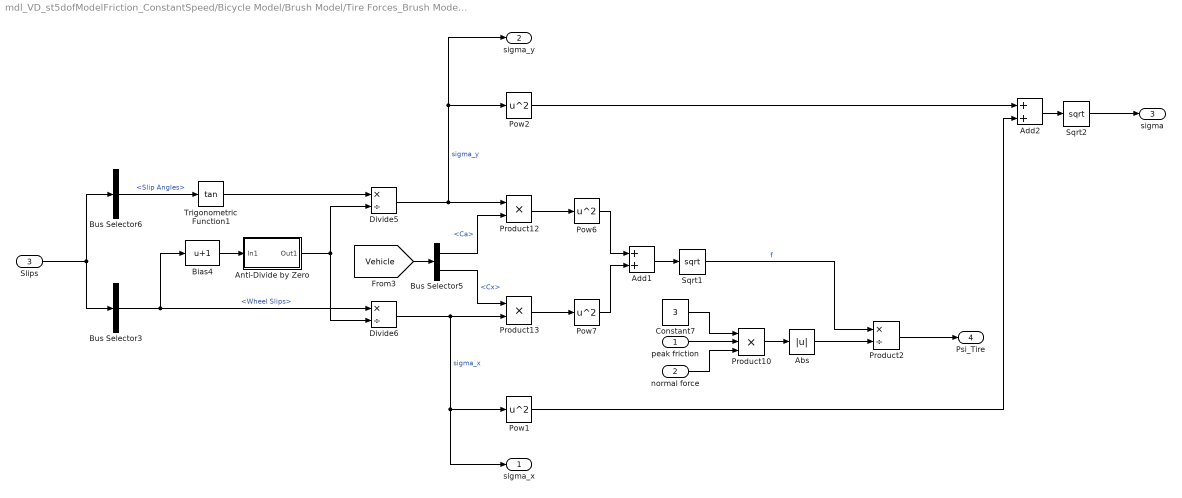
== system mdl_VD_st5dofModelFriction_ConstantSpeed/Bicycle Model/Brush Model/Tire Forces_Brush Model/tire slip ==
  peak friction : Inport
  normal force : Inport  Port=2
  Slips : Inport  Port=3
  Abs : Abs
  Add1 : Sum
  Add2 : Sum
  Anti-Divide by Zero : Subsystem
  Bias4 : Bias  Bias=1
  Bus Selector3 : BusSelector  OutputSignals=Wheel Slips
  Bus Selector5 : BusSelector  OutputSignals=Ca,Cx
  Bus Selector6 : BusSelector  OutputSignals=Slip Angles
  Constant7 : Constant  Value=3
  Divide5 : Product  Inputs=*/
  Divide6 : Product  Inputs=*/
  Pow{1..2,6..7} (4 alike) : Math  Operator=square  SaturateOnIntegerOverflow=on
  Product10 : Product  Inputs=3  RndMeth=Zero
  Product12 : Product  RndMeth=Zero
  Product13 : Product  RndMeth=Zero
  Product2 : Product  Inputs=*/  RndMeth=Zero
  Sqrt1 : Sqrt  SaturateOnIntegerOverflow=on
  Sqrt2 : Sqrt  SaturateOnIntegerOverflow=on
  Trigonometric Function1 : Trigonometry  Operator=tan
  sigma_x : Outport
  sigma_y : Outport  Port=2
  sigma : Outport  Port=3
  Psi_Tire : Outport  Port=4
  wires:
  Sqrt2/1 -> sigma/1
  Pow7/1 -> Add1/2
  Slips/1 -> Bus Selector6/1, Bus Selector3/1
  normal force/1 -> Product10/3
  Product12/1 -> Pow6/1
  Sqrt1/1 -> Product2/1  "f"
  Bus Selector5/2 -> Product13/1  "<Cx>"
  Pow2/1 -> Add2/1
  peak friction/1 -> Product10/2
  Product10/1 -> Abs/1
  Anti-Divide by Zero/1(Out1) -> Divide6/2, Divide5/2
  Constant7/1 -> Product10/1
  Pow1/1 -> Add2/2
  Trigonometric Function1/1 -> Divide5/1
  Add2/1 -> Sqrt2/1
  Divide6/1 -> sigma_x/1, Pow1/1, Product13/2  "sigma_x"
  Product13/1 -> Pow7/1
  Bus Selector3/1 -> Divide6/1, Bias4/1  "<Wheel Slips>"
  Pow6/1 -> Add1/1
  Divide5/1 -> sigma_y/1, Pow2/1, Product12/1  "sigma_y"
  Product2/1 -> Psi_Tire/1
  [Vehicle] -> Bus Selector5/1
  Bus Selector6/1 -> Trigonometric Function1/1  "<Slip Angles>"
  Bias4/1 -> Anti-Divide by Zero/1(In1)
  Bus Selector5/1 -> Product12/2  "<Ca>"
  Add1/1 -> Sqrt1/1
  Abs/1 -> Product2/2

== system mdl_VD_st5dofModelFriction_ConstantSpeed/Bicycle Model/Slips/Wheel Slip Ratio/Wheel Slip ==
  note: κ>0, acceleration→ positive Fx
      | κ<0, braking → negative Fx
  Vx_tire : Inport
  Speeds : Inport  Port=2
  Anti-Divide by Zero : Subsystem
  Bus Selector2 : BusSelector  OutputSignals=Re
  Bus Selector4 : BusSelector  OutputSignals=omega
  Divide2 : Product  Inputs=/*
  Product2 : Product  RndMeth=Zero
  Saturation : Saturate  UpperLimit=1  LowerLimit=-1  ZeroCross=off
  Subtract2 : Sum  Inputs=-+
  Switch1 : Switch  Criteria=u2 > Threshold  ZeroCross=off  SaturateOnIntegerOverflow=on
  Terminator : Terminator
  zero Wheel Slip : Constant  Value=[0 0]
  zero Wheel Slip1 : Constant  Value=[0 0]  SampleTime=-1
  Wheel Slips : Outport
  wires:
  Subtract2/1 -> Divide2/2
  Anti-Divide by Zero/1(Out1) -> Divide2/1
  zero Wheel Slip/1 -> Switch1/3
  Vx_tire/1 -> Anti-Divide by Zero/1(In1), Subtract2/1, Switch1/2
  Bus Selector2/1 -> Product2/2  "<Re>"
  [Vehicle] -> Bus Selector2/1
  Divide2/1 -> Switch1/1
  Switch1/1 -> Saturation/1
  Product2/1 -> Subtract2/2
  zero Wheel Slip1/1 -> Wheel Slips/1  "Wheel Slips"
  Bus Selector4/1 -> Product2/1  "<omega>"
  Speeds/1 -> Bus Selector4/1
  Saturation/1 -> Terminator/1  "Wheel Slips"

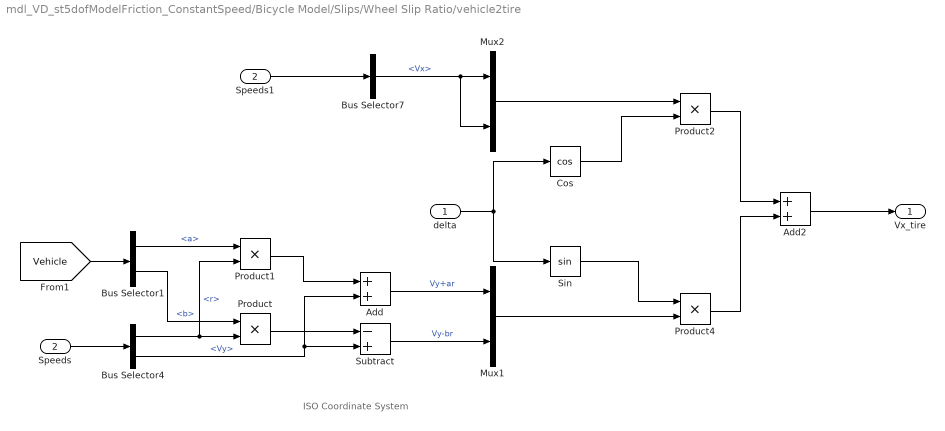
== system mdl_VD_st5dofModelFriction_ConstantSpeed/Bicycle Model/Slips/Wheel Slip Ratio/vehicle2tire ==
  note: ISO Coordinate System
  delta : Inport
  Speeds : Inport  Port=2
  Add : Sum
  Add2 : Sum
  Bus Selector1 : BusSelector  OutputSignals=a,b
  Bus Selector4 : BusSelector  OutputSignals=r,Vy
  Bus Selector7 : BusSelector  OutputSignals=Vx
  Cos : Trigonometry  Operator=cos
  Mux1 : Mux  Inputs=2
  Mux2 : Mux  Inputs=2
  Product{,1..2,4} (4 alike) : Product  RndMeth=Zero
  Sin : Trigonometry
  Speeds1 : InportShadow  Port=2
  Subtract : Sum  Inputs=-+
  Vx_tire : Outport
  wires:
  Speeds1/1 -> Bus Selector7/1
  Bus Selector4/1 -> Product1/2, Product/2  "<r>"
  Bus Selector1/1 -> Product1/1  "<a>"
  Bus Selector7/1 -> Mux2/2, Mux2/1  "<Vx>"
  Product/1 -> Subtract/1
  Bus Selector4/2 -> Add/2, Subtract/2  "<Vy>"
  [Vehicle] -> Bus Selector1/1
  Product1/1 -> Add/1
  Add/1 -> Mux1/1  "Vy+ar"
  Mux2/1 -> Product2/1
  Mux1/1 -> Product4/2
  Bus Selector1/2 -> Product/1  "<b>"
  Speeds/1 -> Bus Selector4/1
  Subtract/1 -> Mux1/2  "Vy-br"
  Product2/1 -> Add2/1
  Add2/1 -> Vx_tire/1
  delta/1 -> Cos/1, Sin/1
  Cos/1 -> Product2/2
  Sin/1 -> Product4/1
  Product4/1 -> Add2/2

== system mdl_VD_st5dofModelFriction_ConstantSpeed/Bicycle Model/Brush Model/Tire Forces_Brush Model/Wheel Forces/Anti-Divide by Zero ==
  In1 : Inport
  Add : Sum
  Compare To Zero : simulink/Logic and Bit Operations/Compare To Zero  relop===  OutDataTypeStr=boolean
  Constant : Constant  Value=eps
  Product : Product
  Out1 : Outport
  wires:
  Add/1 -> Out1/1
  Compare To Zero/1 -> Product/1
  Constant/1 -> Product/2
  Product/1 -> Add/2
  In1/1 -> Compare To Zero/1, Add/1

== system mdl_VD_st5dofModelFriction_ConstantSpeed/Bicycle Model/Brush Model/Tire Forces_Brush Model/tire slip/Anti-Divide by Zero ==
  In1 : Inport
  Add : Sum
  Compare To Zero : simulink/Logic and Bit Operations/Compare To Zero  relop===  OutDataTypeStr=boolean
  Constant : Constant  Value=eps
  Product : Product
  Out1 : Outport
  wires:
  Add/1 -> Out1/1
  Compare To Zero/1 -> Product/1
  Constant/1 -> Product/2
  Product/1 -> Add/2
  In1/1 -> Compare To Zero/1, Add/1

== system mdl_VD_st5dofModelFriction_ConstantSpeed/Bicycle Model/Slips/Wheel Slip Ratio/Wheel Slip/Anti-Divide by Zero ==
  In1 : Inport
  Add : Sum
  Compare To Zero : simulink/Logic and Bit Operations/Compare To Zero  relop===  OutDataTypeStr=boolean
  Constant : Constant  Value=eps
  Product : Product
  Out1 : Outport
  wires:
  In1/1 -> Add/1, Compare To Zero/1
  Product/1 -> Add/2
  Constant/1 -> Product/2
  Compare To Zero/1 -> Product/1
  Add/1 -> Out1/1

== matlab function mdl_VD_st5dofModelFriction_ConstantSpeed/friction estimation/Noise Models/GPS Noise Function ==
  settings: updateMethod=DISCRETE
  data: v_x input; v_x_out output; v_y input; r input; sampling_time input; v_y_out output; r_out output
function [v_x_out, v_y_out, r_out] = GPS_noise(v_x, v_y, r, sampling_time)

% v_x: velocity in X direction [m/s]
% v_y: velocity in Y direction [m/s]
% r: the yaw rate [rad/s]
% sample_rate: frequency at which velocities are being calculated [Hz]

% sensor specifications
sigma_x = 0.025;
sigma_y = 0.025;
sigma_theta = 0.009;

% simulate noisy measurements
v_x_out = v_x + normrnd(0,1.4142*sigma_x)*sampling_time;
v_y_out = v_y + normrnd(0,1.4142*sigma_y)*sampling_time;
r_out   = r + normrnd(0,1.4142*sigma_theta)*sampling_time;

end

== matlab function mdl_VD_st5dofModelFriction_ConstantSpeed/friction estimation/Noise Models/IMU Noise Function ==
  settings: updateMethod=DISCRETE
  data: a_x input; a_x_out output; a_y input; sampling_time input; a_y_out output
function [a_x_out, a_y_out] = IMU_noise(a_x, a_y, sampling_time)

% a_x: accelaration in X direction [m/s^2]
% a_y: accelaration in Y direction [m/s^2]
% alpha: the yaw angular accelaration [rad/s^2]
% sample_rate: frequency at which velocities are being calculated [Hz]

% sensor specifications
sigma_x = 0.25;
sigma_y = 0.25;
% sigma_theta = 0.09;

% simulate noisy measurements
a_x_out = a_x + normrnd(0,2*sigma_x)*(sampling_time^2);
a_y_out = a_y + normrnd(0,2*sigma_y)*(sampling_time^2);
% alpha_out = alpha_in + normrnd(0,2*sigma_theta)*(sampling_time^2);

end
